simulink model "airship_sim"  (R2023b)
settings: Solver=VariableStepAuto  StartTime=0.0  StopTime=1000  FixedStep=1  RelTol=1e-3
undefined symbols (not defined in the file or in its folder): drawSpacecraftBodyVFC
settings Model: Creator=ZuckLee  LastModifiedBy=ZuckLee
settings OptimizationCC: ReuseModelBlockBuffer=off

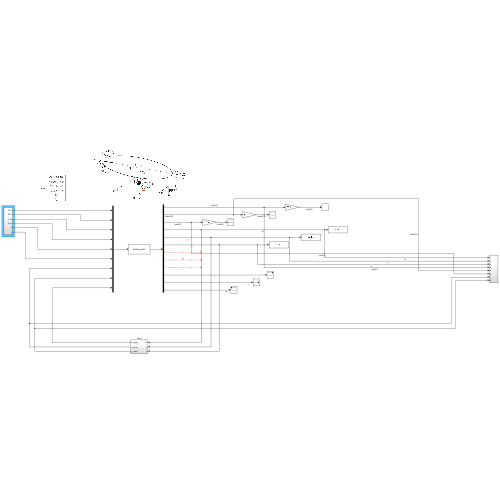
[thumbnail: Simulink's stored preview of the top-level diagram]
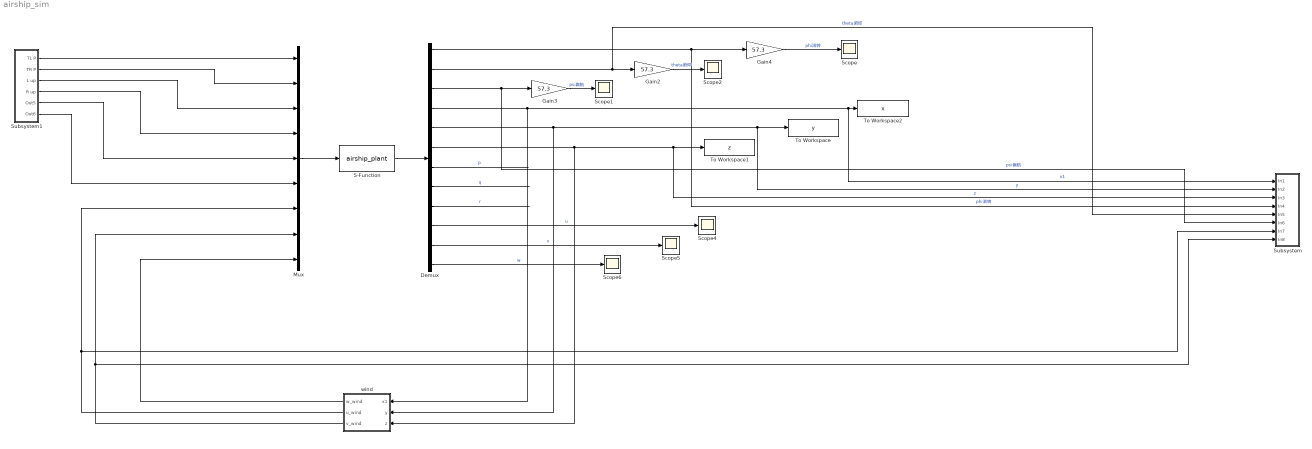
== system airship_sim ==
  Demux : Demux  Outputs=12
  Gain2 : Gain  Gain=57.3
  Gain3 : Gain  Gain=57.3
  Gain4 : Gain  Gain=57.3
  Mux : Mux  Inputs=9
  S-Function : S-Function  FunctionName=airship_plant  SFunctionDeploymentMode=off  EnableBusSupport=off
  Scope{,1..2,4..6} (6 alike) : Scope
  Subsystem : Subsystem
  Subsystem1 : Subsystem
  To Workspace : ToWorkspace  VariableName=y  SampleTime=-1
  To Workspace1 : ToWorkspace  VariableName=z  SampleTime=-1
  To Workspace2 : ToWorkspace  VariableName=x  SampleTime=-1
  wind : Subsystem
  wires:
  S-Function/1 -> Demux/1
  Demux/1 -> Gain4/1, Subsystem/4(In4)  "phi滚转"
  Demux/2 -> Subsystem/5(In5), Gain2/1  "theta俯仰"
  Demux/3 -> Subsystem/6(In6), Gain3/1  "psi偏航"
  Demux/4 -> Subsystem/1(In1), To Workspace2/1, wind/1(x1)  "x1"
  Demux/5 -> Subsystem/2(In2), To Workspace/1, wind/2(y)  "y"
  Demux/6 -> wind/3(z), Subsystem/3(In3), To Workspace1/1  "z"
  Demux/7 -> ?  "p"
  Demux/8 -> ?  "q"
  Demux/9 -> ?  "r"
  Demux/10 -> Scope4/1  "u"
  Demux/11 -> Scope5/1  "v"
  Demux/12 -> Scope6/1  "w"
  Mux/1 -> S-Function/1
  Gain2/1 -> Scope2/1  "theta俯仰"
  Gain3/1 -> Scope1/1  "psi偏航"
  Gain4/1 -> Scope/1  "phi滚转"
  wind/2(u_wind) -> Mux/7, Subsystem/7(In7)
  wind/3(v_wind) -> Mux/8, Subsystem/8(In8)
  wind/1(w_wind) -> Mux/9
  Subsystem1/1(TL P) -> Mux/1
  Subsystem1/2(TR P) -> Mux/2
  Subsystem1/3(L up) -> Mux/3
  Subsystem1/4(R up) -> Mux/4
  Subsystem1/5(Out5) -> Mux/5
  Subsystem1/6(Out6) -> Mux/6

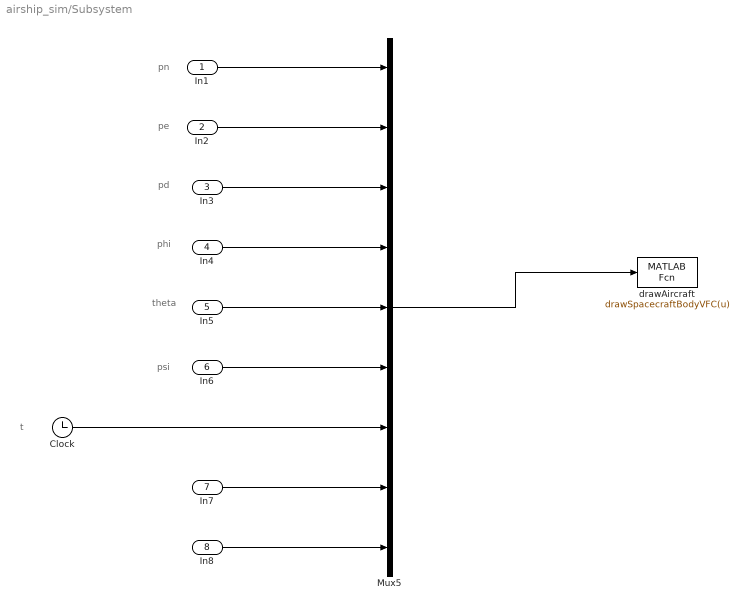
== system airship_sim/Subsystem ==
  note: pd
  note: pe
  note: pn
  note: theta
  note: t
  note: psi
  note: phi
  In1 : Inport
  In2 : Inport  Port=2
  In3 : Inport  Port=3
  In4 : Inport  Port=4
  In5 : Inport  Port=5
  In6 : Inport  Port=6
  In7 : Inport  Port=7
  In8 : Inport  Port=8
  Clock : Clock
  Mux5 : Mux  Inputs=9
  drawAircraft : MATLABFcn  MATLABFcn=drawSpacecraftBodyVFC(u)  OutputDimensions=0  SampleTime=0.1
  wires:
  In6/1 -> Mux5/6
  Mux5/1 -> drawAircraft/1
  Clock/1 -> Mux5/7
  In5/1 -> Mux5/5
  In3/1 -> Mux5/3
  In4/1 -> Mux5/4
  In1/1 -> Mux5/1
  In2/1 -> Mux5/2
  In7/1 -> Mux5/8
  In8/1 -> Mux5/9

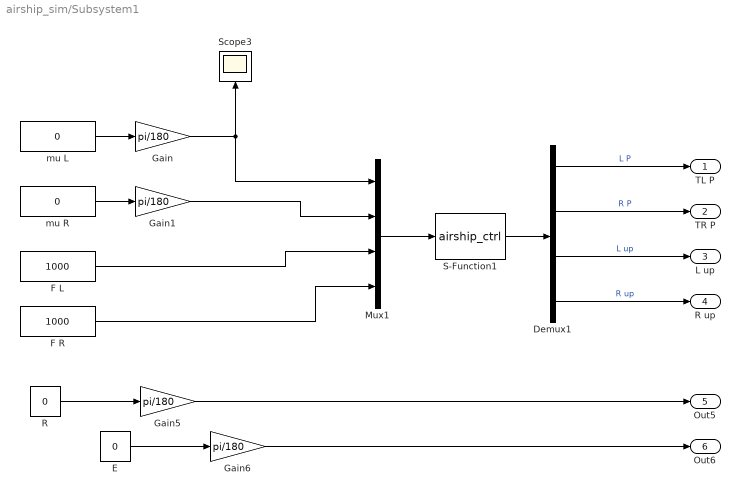
== system airship_sim/Subsystem1 ==
  Demux1 : Demux
  E : Constant  Value=0
  F L : Constant  Value=1000
  F R : Constant  Value=1000
  Gain{,1,5..6} (4 alike) : Gain  Gain=pi/180
  Mux1 : Mux
  R : Constant  Value=0
  S-Function1 : S-Function  FunctionName=airship_ctrl  SFunctionDeploymentMode=off  EnableBusSupport=off
  Scope3 : Scope
  mu L : Constant  Value=0
  mu R : Constant  Value=0
  TL P : Outport
  TR P : Outport  Port=2
  L up : Outport  Port=3
  R up : Outport  Port=4
  Out5 : Outport  Port=5
  Out6 : Outport  Port=6
  wires:
  Gain/1 -> Mux1/1, Scope3/1
  S-Function1/1 -> Demux1/1
  Mux1/1 -> S-Function1/1
  F L/1 -> Mux1/3
  R/1 -> Gain5/1
  E/1 -> Gain6/1
  mu L/1 -> Gain/1
  mu R/1 -> Gain1/1
  Gain1/1 -> Mux1/2
  F R/1 -> Mux1/4
  Demux1/3 -> L up/1  "L up"
  Demux1/1 -> TL P/1  "L P"
  Gain6/1 -> Out6/1
  Demux1/4 -> R up/1  "R up"
  Demux1/2 -> TR P/1  "R P"
  Gain5/1 -> Out5/1

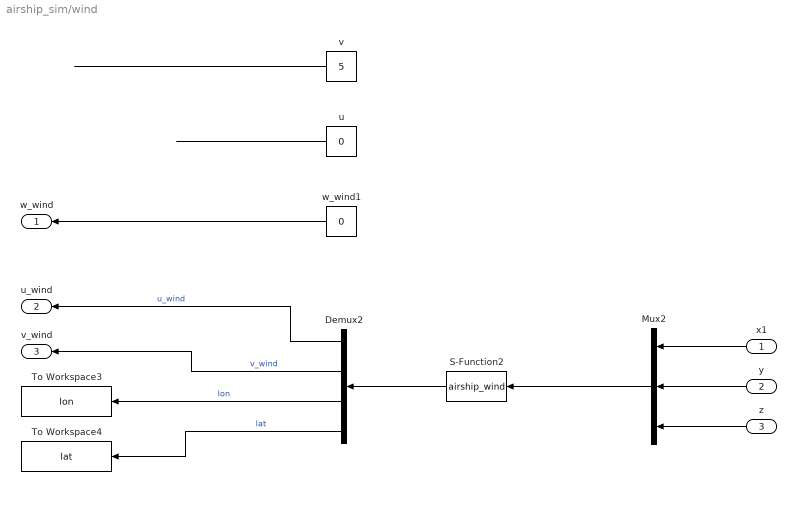
== system airship_sim/wind ==
  x1 : Inport
  y : Inport  Port=2
  z : Inport  Port=3
  Demux2 : Demux
  Mux2 : Mux  Inputs=3
  S-Function2 : S-Function  FunctionName=airship_wind  Parameters=Lat, Lon, u_wind_selected, v_wind_selected  SFunctionDeploymentMode=off  EnableBusSupport=off
  To Workspace3 : ToWorkspace  VariableName=lon  SampleTime=-1
  To Workspace4 : ToWorkspace  VariableName=lat  SampleTime=-1
  u : Constant  Value=0
  v : Constant  Value=5
  w_wind1 : Constant  Value=0
  w_wind : Outport
  u_wind : Outport  Port=2
  v_wind : Outport  Port=3
  wires:
  Mux2/1 -> S-Function2/1
  Demux2/4 -> To Workspace4/1  "lat"
  Demux2/1 -> u_wind/1  "u_wind"
  z/1 -> Mux2/3
  Demux2/2 -> v_wind/1  "v_wind"
  S-Function2/1 -> Demux2/1
  Demux2/3 -> To Workspace3/1  "lon"
  y/1 -> Mux2/2
  x1/1 -> Mux2/1
  w_wind1/1 -> w_wind/1
  u/1 -> ?
  v/1 -> ?
